simulink library "sixDoFKinematics_ul"  (R2018b)
settings: Solver=VariableStepAuto  StartTime=0.0  StopTime=10.0  RelTol=1e-3
undefined symbols (not defined in the file): initAngRates, Jinv
libraries: vrlib x2
settings Model: Creator=mcobb  LastModifiedBy=M.Cobb

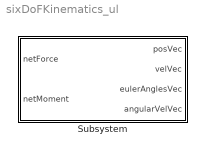
== system sixDoFKinematics_ul ==
  Subsystem : Subsystem  mask{m=1, initPos=0, initVel=0, J=eye(3), initEulAngs=0, initAngVel=0}
      mask prompts: m "Mass"; initPos "Initial position"; initVel "Initial velocity"; J "Inertia matrix"; initEulAngs "Initial Euler Angles"; initAngVel "Initial Angular Velocity Vec"
      mask init:
      | sixDoFKinematics_init

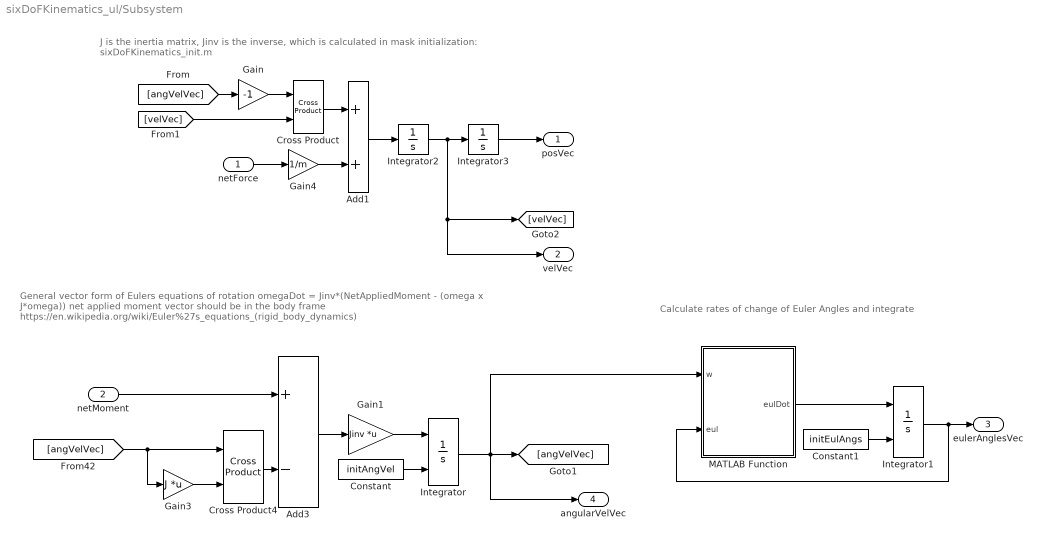
== system sixDoFKinematics_ul/Subsystem ==
  note: Calculate rates of change of Euler Angles and integrate
  note: General vector form of Eulers equations of rotation
      | omegaDot = Jinv*(NetAppliedMoment - (omega x J*omega))
      | net applied moment vector should be in the body frame
      | https://en.wikipedia.org/wiki/Euler%27s_equations_(rigid_body_dynamics)
  note: J is the inertia matrix, Jinv is the inverse, which is calculated in mask initialization: sixDoFKinematics_init.m
  netForce : Inport
  netMoment : Inport  Port=2
  Add1 : Sum
  Add3 : Sum  Inputs=+-
  Constant : Constant  Value=initAngVel
  Constant1 : Constant  Value=initEulAngs
  Cross Product : vrlib/Utilities/Cross Product
      settings: SourceProductBaseCode=VR
  Cross Product4 : vrlib/Utilities/Cross Product
      settings: SourceProductBaseCode=VR
  Gain : Gain  Gain=-1
  Gain1 : Gain  Gain=Jinv  Multiplication=Matrix(K*u)
  Gain3 : Gain  Gain=J  Multiplication=Matrix(K*u)
  Gain4 : Gain  Gain=1/m
  Integrator : Integrator  InitialConditionSource=external  InitialCondition=initAngRates
  Integrator1 : Integrator  InitialConditionSource=external  InitialCondition=initEulAngs
  Integrator2 : Integrator  InitialCondition=initVel
  Integrator3 : Integrator  InitialCondition=initPos
  MATLAB Function : MATLAB Function  TreatAsAtomicUnit=on
  posVec : Outport
  velVec : Outport  Port=2
  eulerAnglesVec : Outport  Port=3
  angularVelVec : Outport  Port=4
  wires:
  netMoment/1 -> Add3/1
  [angVelVec] -> Cross Product4/1, Gain3/1
  Gain3/1 -> Cross Product4/2
  Integrator/1 -> MATLAB Function/1(w), angularVelVec/1, [angVelVec]
  Add3/1 -> Gain1/1
  Integrator1/1 -> MATLAB Function/2(eul), eulerAnglesVec/1
  Gain1/1 -> Integrator/1
  Cross Product4/1 -> Add3/2
  [angVelVec] -> Gain/1
  Gain/1 -> Cross Product/1
  [velVec] -> Cross Product/2
  Cross Product/1 -> Add1/1
  Gain4/1 -> Add1/2
  netForce/1 -> Gain4/1
  Add1/1 -> Integrator2/1
  Integrator3/1 -> posVec/1
  Integrator2/1 -> [velVec], velVec/1, Integrator3/1
  Constant/1 -> Integrator/2
  MATLAB Function/1(eulDot) -> Integrator1/1
  Constant1/1 -> Integrator1/2

== matlab function sixDoFKinematics_ul/Subsystem/MATLAB Function ==
  data: w input; eulDot output; eul input
function eulDot = fcn(w,eul)
% function that relates angular velocity vector to rates of change of Euler
% angles.
% w is angular velocity vector in body frame
% eul is vector of euler angles [roll, pitch, yaw]
eulDot = zeros(3,1);
eulDot(1) = w(1) + sin(eul(1))*tan(eul(2))*w(2) + cos(phi)*tan(eul(2))*w(3);
eulDot(2) = cos(ph)*w(2) - sin(ph)*w(3);...
eulDot(3) = sec(eul(2))*sin(ph)*w(2) + cos(ph)*sec(eul(2))*w(3);
end
